simulink model "LinearSystemPRJsim"  (R2021b)
settings: Solver=VariableStepAuto  StartTime=0.0  StopTime=10.0  RelTol=1e-3
values from neighbouring files (symbols this model uses):
  A = [0 1 0 0 ... (first row only)    [LinearSystemPRJ.m]
  B = [0 0 ... (first row only)    [LinearSystemPRJ.m]
  C = [1 0 0 0 ... (first row only)    [LinearSystemPRJ.m]
  D = zeros(size(C,1),size(B,2))    [LinearSystemPRJ.m]
  G = [g1 g1;g2 g2;g3 g3;g4 g4]    [LinearSystemPRJ.m]
  Kc = place(A,B,P)    [LinearSystemPRJ.m]
settings Model: Creator=MahMooD  LastModifiedBy=MahMooD

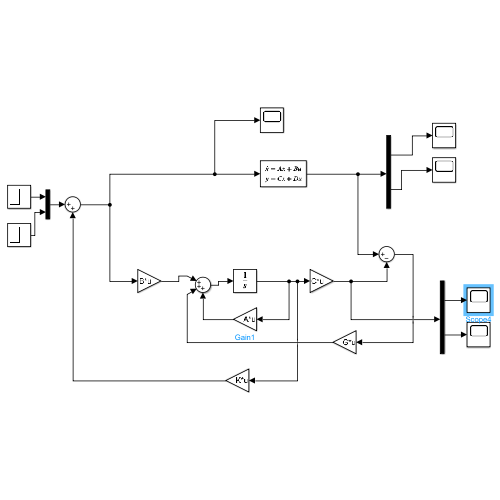
[thumbnail: Simulink's stored preview of the top-level diagram]
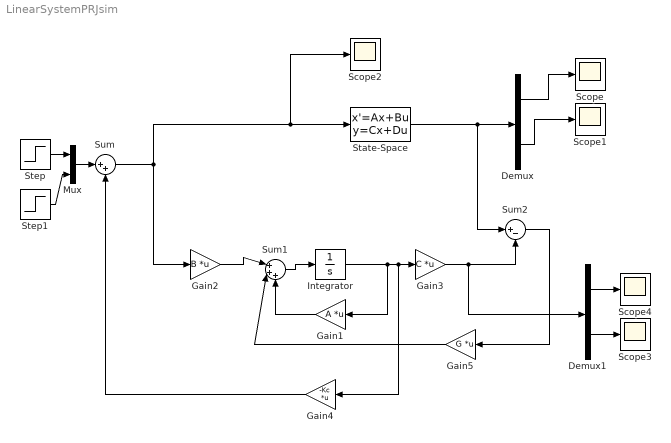
== system LinearSystemPRJsim ==
  Demux : Demux  Outputs=2
  Demux1 : Demux  Outputs=2
  Gain1 : Gain  Gain=A  Multiplication=Matrix(K*u)
  Gain2 : Gain  Gain=B  Multiplication=Matrix(K*u)
  Gain3 : Gain  Gain=C  Multiplication=Matrix(K*u)
  Gain4 : Gain  Gain=-Kc  Multiplication=Matrix(K*u)
  Gain5 : Gain  Gain=G  Multiplication=Matrix(K*u)
  Integrator : Integrator
  Mux : Mux  Inputs=2
  Scope{,1..4} (5 alike) : Scope
  State-Space : StateSpace  A=A  B=B  C=C  D=D  InitialCondition=0  ParameterTunability=Unconstrained
  Step : Step  Time=0  SampleTime=0
  Step1 : Step  Time=0  SampleTime=0
  Sum : Sum  Inputs=|++
  Sum1 : Sum  Inputs=|+++
  Sum2 : Sum  Inputs=|+-
  wires:
  Demux/1 -> Scope/1
  Demux/2 -> Scope1/1
  State-Space/1 -> Sum2/1, Demux/1
  Gain2/1 -> Sum1/1
  Sum1/1 -> Integrator/1
  Gain1/1 -> Sum1/3
  Gain3/1 -> Demux1/1, Sum2/2
  Integrator/1 -> Gain1/1, Gain4/1, Gain3/1
  Sum2/1 -> Gain5/1
  Gain5/1 -> Sum1/2
  Step/1 -> Mux/1
  Step1/1 -> Mux/2
  Mux/1 -> Sum/1
  Gain4/1 -> Sum/2
  Sum/1 -> Scope2/1, State-Space/1, Gain2/1
  Demux1/2 -> Scope3/1
  Demux1/1 -> Scope4/1
